simulink model "Drone_Simulation"  (R2020a)
settings: Solver=ode1  StartTime=0.0  StopTime=50  FixedStep=1e-3
values from neighbouring files (symbols this model uses):
  AeEMSC = 1    [Qball_X8_Model.m]
  alpha1TDDBSC = 1    [Qball_X8_Model.m]    (also in ReliabilityModel_Script.m = 0.7)
  bBNG = 1.2    [ReliabilityModel_Script.m]
  bEMSC = 1    [Qball_X8_Model.m]
  bEVCAP = 1    [Qball_X8_Model.m]    (also in ReliabilityModel_Script.m = 1.1)
  BNG_Motor1 = 0.8    [ReliabilityModel_Script.m]
  BNG_Motor2 = 1    [ReliabilityModel_Script.m]
  BNG_Motor3 = 1    [ReliabilityModel_Script.m]
  BNG_Motor4 = 1    [ReliabilityModel_Script.m]
  BNG_Motor5 = 1    [ReliabilityModel_Script.m]
  BNG_Motor6 = 1    [ReliabilityModel_Script.m]
  bp = 0.001    [ControlLawsScript.m]    (also in ControlLaws_Script.m)
  bq = 0.001    [ControlLawsScript.m]    (also in ControlLaws_Script.m)
  br = 0.001    [ControlLawsScript.m]    (also in ControlLaws_Script.m)
  bTDDBSC = 1    [Qball_X8_Model.m]    (also in ReliabilityModel_Script.m = 1.1)
  bWDG = 1    [Qball_X8_Model.m]    (also in ReliabilityModel_Script.m = 1.1)
  C_A = [     k_T           k_T          k_T                k_T          k_T         k_T ... (first row only)    [ControlLawsScript.m]    (also in ControlLaws_Script.m)
  C_mot = 1    [Qball_X8_Model.m]    (also in ReliabilityModel_Script.m = 17.46)
  C_th_esc = 1    [Qball_X8_Model.m]    (also in ReliabilityModel_Script.m = 1.67)
  CAPEV_Motor1 = 0.8    [ReliabilityModel_Script.m]
  CAPEV_Motor2 = 1    [ReliabilityModel_Script.m]
  CAPEV_Motor3 = 1    [ReliabilityModel_Script.m]
  CAPEV_Motor4 = 1    [ReliabilityModel_Script.m]
  CAPEV_Motor5 = 1    [ReliabilityModel_Script.m]
  CAPEV_Motor6 = 1    [ReliabilityModel_Script.m]
  cdx = cx*m    (= 17.4057414746)    [ControlLawsScript.m]    (also in ControlLaws_Script.m)
  cdy = cy*m    (= 17.4057414746)    [ControlLawsScript.m]    (also in ControlLaws_Script.m)
  cdz = cz*m    (= 17.4057414746)    [ControlLawsScript.m]    (also in ControlLaws_Script.m)
  EaEMSC = 1    [Qball_X8_Model.m]
  EaEVCAP = 1    [Qball_X8_Model.m]    (also in ReliabilityModel_Script.m = 0.94)
  EalphaTDDBSC = 1    [Qball_X8_Model.m]    (also in ReliabilityModel_Script.m = 0.7)
  EaTDDBSC = 1    [Qball_X8_Model.m]    (also in ReliabilityModel_Script.m = 0.7)
  EaWDG = 1    [Qball_X8_Model.m]    (also in ReliabilityModel_Script.m = 0.5)
  g = 9.80665    [ControlLawsScript.m]    (also in ControlLaws_Script.m; Qball_X8_Model.m = 9.87)
  JrefEMSC = 1    [Qball_X8_Model.m]
  Jz = 0.15887270137511    (= 0.158872701375)    [ControlLawsScript.m]    (also in ControlLaws_Script.m)
  k_b = 1    [Qball_X8_Model.m]    (also in ReliabilityModel_Script.m = -21.8546)
  Kp = (Jx/Tc)-bp    (= 4.11390529802)    [ControlLawsScript.m]    (also in ControlLaws_Script.m)
  Kp2 = Jx*((4/ts))*((-4/ts)+((bp+Kp)/Jx))/Kp    (= 6.72163348437)    [ControlLawsScript.m]    (also in ControlLaws_Script.m)
  Kq = (Jy/Tc)-bq    (= 4.12186008142)    [ControlLawsScript.m]    (also in ControlLaws_Script.m)
  Kq2 = Jy*((4/ts))*((-4/ts)+((bq+Kq)/Jy))/Kq    (= 6.72163033191)    [ControlLawsScript.m]    (also in ControlLaws_Script.m)
  Kr = (Jz/(tsy/25))-br    (= 7.94263506876)    [ControlLawsScript.m]    (also in ControlLaws_Script.m)
  Kr2 = Jz*((4/tsy))*((-4/tsy)+((br+Kr)/Jz))/Kr    (= 6.72084606682)    [ControlLawsScript.m]    (also in ControlLaws_Script.m)
  kv = 1/930    (= 0.0010752688172)    [StingerScript.m]
  Kx = abs(Kx)    [ControlLawsScript.m]    (also in ControlLaws_Script.m)
  Ky = abs(Ky)    [ControlLawsScript.m]    (also in ControlLaws_Script.m)
  Kz = (m/Tcz)-cz    (= 38.5143536865)    [ControlLawsScript.m]    (also in ControlLaws_Script.m)
  Kz2 = m*((4/tsz))*((-4/tsz)+((cz+Kz)/m))/Kz    (= 1.89810050529)    [ControlLawsScript.m]    (also in ControlLaws_Script.m)
  LnomEMSC = 1    [Qball_X8_Model.m]
  LnomEVCAP = 1    [Qball_X8_Model.m]    (also in ReliabilityModel_Script.m = 10800000)
  LnomTDDBSC = 1    [Qball_X8_Model.m]    (also in ReliabilityModel_Script.m = 9997200)
  LnomWDG = 1    [Qball_X8_Model.m]    (also in ReliabilityModel_Script.m = 72000000)
  m = 3.4811482949175    (= 3.48114829492)    [ControlLawsScript.m]    (also in ControlLaws_Script.m; Qball_X8_Model.m = 1.45)
  max_yaw_moment = k_y*hov_thrust/k_T    (= 0.323744079512)    [ControlLawsScript.m]    (also in ControlLaws_Script.m = 0.57666914163)
  NEMSC = 1    [Qball_X8_Model.m]
  nEVCAP = 1    [Qball_X8_Model.m]    (also in ReliabilityModel_Script.m)
  pconst = 2    [Qball_X8_Model.m]    (also in ReliabilityModel_Script.m)
  pitch_angle_limit = 32/R2D    (= 0.558505360638)    [ControlLawsScript.m]    (also in ControlLaws_Script.m)
  R2D = 180/pi    (= 57.2957795131)    [ControlLawsScript.m]    (also in ControlLaws_Script.m)
  R_th_esc = 1    [Qball_X8_Model.m]    (also in ReliabilityModel_Script.m = 5.14)
  R_th_mot = 1    [Qball_X8_Model.m]    (also in ReliabilityModel_Script.m = 8.59)
  Re = 0.008    [Qball_X8_Model.m]    (also in ReliabilityModel_Script.m)
  roll_angle_limit = 32/R2D    (= 0.558505360638)    [ControlLawsScript.m]    (also in ControlLaws_Script.m)
  RrefBNG = 0.9    [ReliabilityModel_Script.m]
  RrefEMSC = 1    [Qball_X8_Model.m]
  RrefEVCAP = 1    [Qball_X8_Model.m]    (also in ReliabilityModel_Script.m = 0.9)
  RrefTDDBSC = 1    [Qball_X8_Model.m]    (also in ReliabilityModel_Script.m = 0.37)
  RrefWDG = 1    [Qball_X8_Model.m]    (also in ReliabilityModel_Script.m = 0.98)
  SCTDDB_Motor1 = 0.8    [ReliabilityModel_Script.m]
  SCTDDB_Motor2 = 1    [ReliabilityModel_Script.m]
  SCTDDB_Motor3 = 1    [ReliabilityModel_Script.m]
  SCTDDB_Motor4 = 1    [ReliabilityModel_Script.m]
  SCTDDB_Motor5 = 1    [ReliabilityModel_Script.m]
  SCTDDB_Motor6 = 1    [ReliabilityModel_Script.m]
  T_amb = 1    [Qball_X8_Model.m]    (also in ReliabilityModel_Script.m = 20)
  T_amb_mot = 1    [Qball_X8_Model.m]    (also in ReliabilityModel_Script.m = 20)
  t_D_SCTDDB = 30    [ReliabilityModel_Script.m]
  TrefEMSC = 1    [Qball_X8_Model.m]
  TrefEVCAP = 1    [Qball_X8_Model.m]    (also in ReliabilityModel_Script.m = 105)
  TrefTDDBSC = 1    [Qball_X8_Model.m]    (also in ReliabilityModel_Script.m = 150)
  TrefWDG = 1    [Qball_X8_Model.m]    (also in ReliabilityModel_Script.m = 40)
  Ub = 12    [Qball_X8_Model.m]    (also in ReliabilityModel_Script.m)
  VmaxEVCAP = 1    [Qball_X8_Model.m]    (also in ReliabilityModel_Script.m = 35)
  VnomEVCAP = 1    [Qball_X8_Model.m]    (also in ReliabilityModel_Script.m = 35)
  WDG_Motor1 = 0.8    [ReliabilityModel_Script.m]
  WDG_Motor2 = 1    [ReliabilityModel_Script.m]
  WDG_Motor3 = 1    [ReliabilityModel_Script.m]
  WDG_Motor4 = 1    [ReliabilityModel_Script.m]
  WDG_Motor5 = 1    [ReliabilityModel_Script.m]
  WDG_Motor6 = 1    [ReliabilityModel_Script.m]
  z_x = cx    (= 5)    [ControlLawsScript.m]    (also in ControlLaws_Script.m)
  z_y = cy    (= 5)    [ControlLawsScript.m]    (also in ControlLaws_Script.m)
undefined symbols (not defined in the file or in its folder): FuselageContactForces, LeftAftArm, LeftAftSkid, LeftArm, LeftFrontArm, LeftFrontSkid, LeftSideContactForces, Lower, missionPlanX, missionPlanY, missionPlanYaw, missionPlanZ, Newton, Raphson, RightAftArm, RightAftSkid, RightArm, RightFrontArm, RightFrontSkid, RightSideContactForces, SkidsContactForces, timeConstant, Upper, X, Y, Z
libraries: sm_lib x90, nesl_utility x78, fl_lib x61, ee_lib x19, dspinverses x1, dspmtrx3 x1
(part 2 of 5)

== system Drone_Simulation/CONTROL ALLOCATION/Reliability Observer (SCTDDB)1 ==
  T_IN : Inport
  V_ESC_OUT : Inport  Port=2
  Cumulative Aging VTDDB : Subsystem
  LambdaTDDB : Subsystem
  ReliabilityTDDB : Subsystem
  VrefTDDB : Subsystem
  R_RT_SCTDDB : Outport
  LambdaSCTDDB : Outport  Port=2
  wires:
  V_ESC_OUT/1 -> Cumulative Aging VTDDB/2(V_ESC_OUT)
  LambdaTDDB/1(Out1) -> LambdaSCTDDB/1
  ReliabilityTDDB/1(Out1) -> R_RT_SCTDDB/1
  Cumulative Aging VTDDB/1(Out1) -> LambdaTDDB/1(In1), ReliabilityTDDB/1(In1)
  VrefTDDB/1(Out1) -> LambdaTDDB/2(In2), ReliabilityTDDB/2(In2)
  T_IN/1 -> Cumulative Aging VTDDB/1(T_IN)

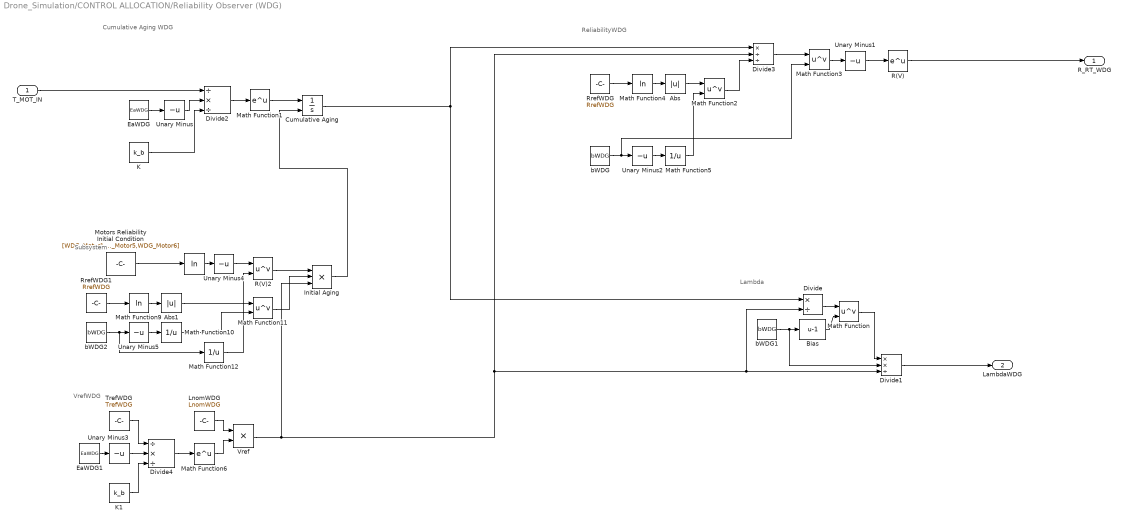
== system Drone_Simulation/CONTROL ALLOCATION/Reliability Observer (WDG) ==
  note: Lambda
  note: ReliabilityWDG
  note: VrefWDG
  note: Cumulative Aging WDG
  note: Subsystem
  T_MOT_IN : Inport
  " " : Math  Operator=log  SaturateOnIntegerOverflow=on
  Abs : Abs
  Abs1 : Abs
  Bias : Bias  Bias=-1
  Cumulative Aging : Integrator  InitialConditionSource=external
  Divide : Product  Inputs=*/
  Divide1 : Product  Inputs=**/
  Divide2 : Product  Inputs=/*/
  Divide3 : Product  Inputs=*//
  Divide4 : Product  Inputs=/*/
  EaWDG : Constant  Value=EaWDG
  EaWDG1 : Constant  Value=EaWDG
  Initial Aging : Product  Inputs=3
  K : Constant  Value=k_b
  K1 : Constant  Value=k_b
  LnomWDG : Constant  Value=LnomWDG
  Math Function{,2..3,11} (4 alike) : Math  Operator=pow  SaturateOnIntegerOverflow=on
  Math Function1 : Math  SaturateOnIntegerOverflow=on
  Math Function10 : Math  Operator=reciprocal  SaturateOnIntegerOverflow=on
  Math Function12 : Math  Operator=reciprocal  SaturateOnIntegerOverflow=on
  Math Function4 : Math  Operator=log  SaturateOnIntegerOverflow=on
  Math Function5 : Math  Operator=reciprocal  SaturateOnIntegerOverflow=on
  Math Function6 : Math  SaturateOnIntegerOverflow=on
  Math Function9 : Math  Operator=log  SaturateOnIntegerOverflow=on
  Motors Reliability Initial Condition : Constant  Value=[WDG_Motor1,WDG_Motor2,WDG_Motor3,WDG_Motor4,WDG_Motor5,WDG_Motor6]
  R(V) : Math  SaturateOnIntegerOverflow=on
  R(V)2 : Math  Operator=pow  SaturateOnIntegerOverflow=on
  RrefWDG : Constant  Value=RrefWDG
  RrefWDG1 : Constant  Value=RrefWDG
  TrefWDG : Constant  Value=TrefWDG
  Unary Minus{,1..5} (6 alike) : UnaryMinus
  Vref : Product
  bWDG : Constant  Value=bWDG
  bWDG1 : Constant  Value=bWDG
  bWDG2 : Constant  Value=bWDG
  R_RT_WDG : Outport
  LambdaWDG : Outport  Port=2
  wires:
  Divide1/1 -> LambdaWDG/1
  R(V)/1 -> R_RT_WDG/1
  T_MOT_IN/1 -> Divide2/1
  Unary Minus/1 -> Divide2/2
  Divide2/1 -> Math Function1/1
  K/1 -> Divide2/3
  EaWDG/1 -> Unary Minus/1
  Math Function1/1 -> Cumulative Aging/1
  TrefWDG/1 -> Divide4/1
  Divide4/1 -> Math Function6/1
  Math Function6/1 -> Vref/2
  LnomWDG/1 -> Vref/1
  K1/1 -> Divide4/3
  Unary Minus3/1 -> Divide4/2
  EaWDG1/1 -> Unary Minus3/1
  Unary Minus2/1 -> Math Function5/1
  Math Function2/1 -> Divide3/3
  RrefWDG/1 -> Math Function4/1
  Math Function5/1 -> Math Function2/2
  Math Function3/1 -> Unary Minus1/1
  bWDG/1 -> Math Function3/2, Unary Minus2/1
  Unary Minus1/1 -> R(V)/1
  Math Function4/1 -> Abs/1
  Abs/1 -> Math Function2/1
  Divide3/1 -> Math Function3/1
  Cumulative Aging/1 -> Divide3/1, Divide/1
  Divide/1 -> Math Function/1
  bWDG1/1 -> Divide1/2, Bias/1
  Math Function/1 -> Divide1/1
  Bias/1 -> Math Function/2
  Vref/1 -> Divide3/2, Divide/2, Divide1/3, Initial Aging/3
  Initial Aging/1 -> Cumulative Aging/2
  Math Function12/1 -> R(V)2/2
  Math Function10/1 -> Math Function11/2
  R(V)2/1 -> Initial Aging/1
  Math Function9/1 -> Abs1/1
  Abs1/1 -> Math Function11/1
  RrefWDG1/1 -> Math Function9/1
  bWDG2/1 -> Math Function12/1, Unary Minus5/1
  " "/1 -> Unary Minus4/1
  Unary Minus4/1 -> R(V)2/1
  Motors Reliability Initial Condition/1 -> " "/1
  Math Function11/1 -> Initial Aging/2
  Unary Minus5/1 -> Math Function10/1

== system Drone_Simulation/CONTROL ALLOCATION/Reliability Observer (WDG)1 ==
  T_MOT_IN : Inport
  Cumulative Aging WDG : Subsystem
  Display : Display
  Lambda : Subsystem
  ReliabilityWDG : Subsystem
  VrefWDG : Subsystem
  R_RT_WDG : Outport
  LambdaWDG : Outport  Port=2
  wires:
  ReliabilityWDG/1(Out1) -> R_RT_WDG/1
  T_MOT_IN/1 -> Cumulative Aging WDG/1(In1)
  Cumulative Aging WDG/1(Out1) -> ReliabilityWDG/1(In1), Lambda/1(In1), Display/1
  VrefWDG/1(Out1) -> ReliabilityWDG/2(In2), Lambda/2(In2)
  Lambda/1(Out1) -> LambdaWDG/1

== system Drone_Simulation/CONTROL ALLOCATION/Thermal Model (ESC)2 ==
  note: Will update, temporary values ->
  V_ESC_in (V) : Inport  PortDimensions=6
  I_ESC_in (A) : Inport  Port=2  PortDimensions=6
  V_ESC_OUT : Inport  Port=3
  I_ESC_OUT : Inport  Port=4
  Demux : Demux  Outputs=6
  Display : Display
  Mux : Mux  Inputs=6
      settings: DisplayOption=signals
  Product : Product
  Product1 : Product
  Product2 : Product
  R_th_esc : Constant  Value=[R_th_esc;R_th_esc;R_th_esc;R_th_esc;R_th_esc;R_th_esc]
  Saturation : Saturate  UpperLimit=400  LowerLimit=T_amb
  Subtract : Sum  Inputs=+-
  Subtract1 : Sum
  T_amb : Constant  Value=[T_amb;T_amb;T_amb;T_amb;T_amb;T_amb]
  Transfer Fcn{,1..5} (6 alike) : TransferFcn  Denominator=[R_th_esc*C_th_esc 1]
  T_ESC_IN : Outport
  wires:
  V_ESC_in (V)/1 -> Product/1
  I_ESC_in (A)/1 -> Product/2
  Product/1 -> Subtract/1
  Product2/1 -> Subtract/2
  Subtract/1 -> Product1/1
  R_th_esc/1 -> Product1/2
  Product1/1 -> Subtract1/1
  V_ESC_OUT/1 -> Product2/1
  I_ESC_OUT/1 -> Product2/2
  Subtract1/1 -> Demux/1
  Transfer Fcn5/1 -> Mux/6
  Transfer Fcn1/1 -> Mux/2
  Transfer Fcn4/1 -> Mux/5
  Transfer Fcn/1 -> Mux/1
  Transfer Fcn3/1 -> Mux/4
  Demux/1 -> Transfer Fcn/1
  Transfer Fcn2/1 -> Mux/3
  Demux/3 -> Transfer Fcn2/1
  Demux/6 -> Transfer Fcn5/1
  Demux/5 -> Transfer Fcn4/1
  Demux/4 -> Transfer Fcn3/1
  Demux/2 -> Transfer Fcn1/1
  T_amb/1 -> Subtract1/2
  Saturation/1 -> Display/1, T_ESC_IN/1
  Mux/1 -> Saturation/1

== system Drone_Simulation/CONTROL ALLOCATION/Thermal Model (Motor)2 ==
  Torque : Inport  PortDimensions=6
  RPM : Inport  Port=2  PortDimensions=6
  V_ESC_OUT : Inport  Port=3  PortDimensions=6
  I_ESC_OUT : Inport  Port=4  PortDimensions=6
  Delay : Delay
  Demux : Demux  Outputs=6
  Display : Display
  Display1 : Display
  Display2 : Display
  Gain : Gain  Gain=pi/180
  Mux : Mux  Inputs=6
  Product : Product
  Product1 : Product
  Product2 : Product
  R_th_mot : Constant  Value=[R_th_mot;R_th_mot;R_th_mot;R_th_mot;R_th_mot;R_th_mot]
  Saturation : Saturate  UpperLimit=400  LowerLimit=T_amb_mot
  Subtract : Sum  Inputs=+-
  Subtract1 : Sum
  T_amb_mot : Constant  Value=[T_amb_mot;T_amb_mot;T_amb_mot;T_amb_mot;T_amb_mot;T_amb_mot]
  Transfer Fcn{,1..5} (6 alike) : TransferFcn  Denominator=[R_th_mot*C_mot 1]
  T_MOT_IN : Outport  PortDimensions=6
  wires:
  Subtract/1 -> Product1/1
  R_th_mot/1 -> Product1/2
  Product1/1 -> Subtract1/1, Display/1
  T_amb_mot/1 -> Display1/1, Subtract1/2
  Product2/1 -> Subtract/1
  Product/1 -> Subtract/2
  Torque/1 -> Product/1
  I_ESC_OUT/1 -> Product2/2
  V_ESC_OUT/1 -> Delay/1
  Subtract1/1 -> Demux/1
  Demux/1 -> Transfer Fcn/1
  Demux/2 -> Transfer Fcn1/1
  Demux/4 -> Transfer Fcn3/1
  Demux/3 -> Transfer Fcn2/1
  Demux/5 -> Transfer Fcn4/1
  Demux/6 -> Transfer Fcn5/1
  Transfer Fcn/1 -> Mux/1
  Transfer Fcn1/1 -> Mux/2
  Transfer Fcn3/1 -> Mux/4
  Transfer Fcn4/1 -> Mux/5
  Mux/1 -> Saturation/1, Display2/1
  Gain/1 -> Product/2
  RPM/1 -> Gain/1
  Transfer Fcn2/1 -> Mux/3
  Transfer Fcn5/1 -> Mux/6
  Delay/1 -> Product2/1
  Saturation/1 -> T_MOT_IN/1

== system Drone_Simulation/PLANT MODEL/BODY ==
  Lower Body : sm_lib/Body Elements/File Solid  ExtGeomFileName=STL files\LowerBody.stl  UnitType=Custom  ExtGeomFileUnits=mm  StepReaderType=HEX  ExportConvexHullGeometry=on  InertiaType=CalculateFromGeometry  Mass=1.038628  MassUnits=kg  CenterOfMass=[0, 0, -1.64462e-2]  CenterOfMassUnits=m  MomentsOfInertia=[5.66226e-3 5.662277e-3 1.11925e-2]  MomentsOfInertiaUnits=kg*m^2  ProductsOfInertia=[0 0 6.64514e-10]  ProductsOfInertiaUnits=kg*m^2  BasedOnType=Density  Density=rho  DensityUnits=kg/m^3  DoExposeReferenceFrame=on  SerializedFrames=<Frames/>  GraphicType=FromGeometry  MarkerShape=Sphere  MarkerSize=10  GraphicVisPropType=SimpleVisualProperties  GraphicDiffuseColor=rgb  GraphicSpecularColor=[0.5 0.5 0.5 1.0]  GraphicAmbientColor=[0.15 0.15 0.15 1.0]  GraphicEmissiveColor=[0.0 0.0 0.0 1.0]  GraphicShininess=75  GraphicOpacity=op
  SKIDS : Subsystem  mask{rho2=788, rgb2=[1 1 1], op2=1}
      mask prompts: rho2 "Density of Skid (kg/m^3)"; rgb2 "Color of Skid [R G B]"; op2 "Opacity of Skid (0-1)"
      mask Display: image('$imagefile'); % Use "Edit Image" on toolstrip to change.
  Simscape Bus : SimscapeBus  HierarchyStrings=Upper;Lower
  Upper Body : sm_lib/Body Elements/File Solid  ExtGeomFileName=STL files\UpperBody.stl  UnitType=Custom  ExtGeomFileUnits=mm  StepReaderType=HEX  ExportConvexHullGeometry=on  InertiaType=CalculateFromGeometry  Mass=1.05986327  MassUnits=kg  CenterOfMass=[0 0 1.6454e-2]  CenterOfMassUnits=m  MomentsOfInertia=[5.7148e-3 5.6834e-3 1.12655e-2]  MomentsOfInertiaUnits=kg*m^2  ProductsOfInertia=[0 0 6.7805e-10]  ProductsOfInertiaUnits=kg*m^2  BasedOnType=Density  Density=rho  DensityUnits=kg/m^3  DoExposeReferenceFrame=on  SerializedFrames=<Frames/>  GraphicType=FromGeometry  MarkerShape=Sphere  MarkerSize=10  GraphicVisPropType=SimpleVisualProperties  GraphicDiffuseColor=rgb  GraphicSpecularColor=[0.5 0.5 0.5 1.0]  GraphicAmbientColor=[0.15 0.15 0.15 1.0]  GraphicEmissiveColor=[0.0 0.0 0.0 1.0]  GraphicShininess=75  GraphicOpacity=op
  Contact : PMIOPort  Side=Left
  Plant : PMIOPort  Port=2  Side=Right
  Contact1 : PMIOPort  Port=3  Side=Left
  connections:
  Upper Body/LConn1 -- Simscape Bus/LConn1
  Upper Body/RConn1 -- Lower Body/RConn1 -- Plant/RConn1 -- SKIDS/LConn2
  Contact/RConn1 -- Simscape Bus/RConn1
  Simscape Bus/LConn2 -- Lower Body/LConn1
  Contact1/RConn1 -- SKIDS/LConn1

== system Drone_Simulation/PLANT MODEL/CONTACT FORCES ==
  Left Contact Arms : SimscapeBus  HierarchyStrings=LeftFrontArm;LeftArm;LeftAftArm
  Right Contact Arms : SimscapeBus  HierarchyStrings=RightFrontArm;RightArm;RightAftArm
  Right Contact Skids : SimscapeBus  HierarchyStrings=LeftAftSkid;LeftFrontSkid;RightFrontSkid;RightAftSkid
  Simscape Bus : SimscapeBus  HierarchyStrings=FuselageContactForces;LeftSideContactForces;RightSideContactForces;SkidsContactForces
  Simscape Bus1 : SimscapeBus  HierarchyStrings=Upper;Lower
  Spatial Contact Force{,1..11} (12 alike) : sm_lib/Forces and Torques/Spatial Contact Force  CoefficientOfDynamicFriction=mud  CoefficientOfStaticFriction=mus  NormalDamping=b  NormalDampingUnits=N/(m/s)  NormalStiffness=st  NormalStiffnessUnits=N/m  FrictionalCriticalVelocity=vcr  FrictionalCriticalVelocityUnits=m/s  ZeroCrossDetectContactStartAndEnd=off  SenseFrictionalForceMagnitude=off  SenseNormalForceMagnitude=off  SenseSeparationDistance=off  NormalTransitionRegionWidth=trans  NormalTransitionRegionWidthUnits=m  FrictionType=SmoothStickSlip
  GC : PMIOPort  Side=Right
  Contact Forces : PMIOPort  Port=2  Side=Right
  connections:
  Spatial Contact Force/RConn1 -- Spatial Contact Force9/RConn1 -- GC/RConn1 -- Spatial Contact Force1/RConn1 -- Spatial Contact Force2/RConn1 -- Spatial Contact Force3/RConn1 -- Spatial Contact Force4/RConn1 -- Spatial Contact Force5/RConn1 -- Spatial Contact Force6/RConn1 -- Spatial Contact Force11/RConn1 -- Spatial Contact Force10/RConn1 -- Spatial Contact Force8/RConn1 -- Spatial Contact Force7/RConn1
  Right Contact Arms/LConn3 -- Spatial Contact Force6/LConn1
  Right Contact Arms/LConn2 -- Spatial Contact Force5/LConn1
  Right Contact Arms/LConn1 -- Spatial Contact Force4/LConn1
  Left Contact Arms/LConn2 -- Spatial Contact Force2/LConn1
  Spatial Contact Force1/LConn1 -- Left Contact Arms/LConn1
  Left Contact Arms/LConn3 -- Spatial Contact Force3/LConn1
  Right Contact Skids/LConn1 -- Spatial Contact Force11/LConn1
  Right Contact Skids/LConn2 -- Spatial Contact Force10/LConn1
  Spatial Contact Force8/LConn1 -- Right Contact Skids/LConn3
  Right Contact Skids/LConn4 -- Spatial Contact Force7/LConn1
  Simscape Bus/LConn2 -- Left Contact Arms/RConn1
  Simscape Bus/LConn3 -- Right Contact Arms/RConn1
  Simscape Bus/LConn4 -- Right Contact Skids/RConn1
  Contact Forces/RConn1 -- Simscape Bus/RConn1
  Simscape Bus1/RConn1 -- Simscape Bus/LConn1
  Spatial Contact Force/LConn1 -- Simscape Bus1/LConn2
  Spatial Contact Force9/LConn1 -- Simscape Bus1/LConn1

== system Drone_Simulation/PLANT MODEL/DRAG FORCES ==
  note: Drag Constants
  External Force and Torque : sm_lib/Forces and Torques/External Force and Torque  ForceResolutionFrame=AttachedFrame  EnableForceX=on  EnableForceY=on  EnableForceZ=on  EnableForce=off  TorqueResolutionFrame=AttachedFrame  EnableTorqueX=on  EnableTorqueY=on  EnableTorqueZ=on  EnableTorque=off
  Gain15 : Gain  Gain=-cdx
  Gain16 : Gain  Gain=-cdy
  Gain17 : Gain  Gain=-cdz
  Gain18 : Gain  Gain=-bq
  Gain19 : Gain  Gain=0
  Gain20 : Gain  Gain=bp
  Simulink-PS Converter{,1..5} (6 alike) : nesl_utility/Simulink-PS Converter  PhysicalDomain=network_engine_domain  SubClassName=ps_input  LeftPortType=input  RightPortType=output  PseudoPeriodic=off  Frequencies=[]  NoiseDistribution=none  NoiseParameters=[]  Unit=1  AffineConversion=off  FilteringAndDerivatives=provide  SimscapeFilterOrder=1  InputFilterTimeConstant=0.001  UdotUserProvided=0
  Model : PMIOPort  Side=Right
  wires:
  Gain20/1 -> Simulink-PS Converter/1  "tx"
  Gain17/1 -> Simulink-PS Converter3/1  "fz"
  Gain15/1 -> Simulink-PS Converter5/1  "fx"
  Gain16/1 -> Simulink-PS Converter4/1  "fy"
  Gain18/1 -> Simulink-PS Converter1/1  "ty"
  Gain19/1 -> Simulink-PS Converter2/1  "tz"
  [DZ] -> Gain17/1
  [DY] -> Gain16/1
  [DX] -> Gain15/1
  [rollAngleSpeed] -> Gain20/1
  [pitchAngleSpeed] -> Gain18/1
  [yawAngleSpeed] -> Gain19/1
  connections:
  Simulink-PS Converter4/RConn1 -- External Force and Torque/LConn2
  Simulink-PS Converter5/RConn1 -- External Force and Torque/LConn1
  Simulink-PS Converter2/RConn1 -- External Force and Torque/LConn6
  Simulink-PS Converter/RConn1 -- External Force and Torque/LConn4
  Simulink-PS Converter1/RConn1 -- External Force and Torque/LConn5
  Simulink-PS Converter3/RConn1 -- External Force and Torque/LConn3
  Model/RConn1 -- External Force and Torque/RConn1

== system Drone_Simulation/PLANT MODEL/ELECTRIC SYSTEM ==
  Battery 1 (Table-Based)1 : ee_lib/Sources/Battery (Table-Based)  Commented=on  SOC_vec=[0,0.05,0.1,0.15,0.2,0.25,0.3,0.35,0.4,0.45,0.5,0.55,0.6,0.65,0.7,0.75,0.8,0.85,0.9,0.95,1]  T_dependence=ee.enum.temperature_dependence.no  T_vec=[273.15, 298.15, 323.15] K  V0_mat=[3.2, 3.1, 3.14; 3.25, 3.27, 3.3; 3.28, 3.31, 3.34; 3.33, 3.5, 3.59] V  V0_vec=[0,12,13,13.4,13.62,13.75,13.85,13.91,13.95,14,14,14,14,14,14,14,14,14,14,14.6,16.8] V  R0_mat=[.03, .015, .002; .04, .017, .008; .039, .012, .006; .027, .013, .021] Ohm  R0_vec=[0.014,0.014,0.014,0.014,0.014,0.014,0.014,0.014,0.014,0.014,0.014,0.014,0.014,0.014,0.014,0.014,0.014,0.014,0.014,0.014,0.014] Ohm  AH_vec=[2.9, 4.1, 4.2] hr*A  AH=5.2 hr*A  prm_leak=ee.enum.battery.prm_leak.disabled  Rleak_vec=[8000, 7000, 6000] Ohm  Rleak=7e3 Ohm  extrapolation_option=ee.enum.extrapolation.nearest  prm_dyn=ee.enum.battery.prm_dyn.off  R1_mat=[.089, .076, .01; .042, .022, .099; .019, .007, .002; .051, .043, .029] Ohm  R1_vec=[.076, .022, .007, .043] Ohm  tau1_mat=[44, 148, 235; 93, 110, 1000; 19, 27, 133; .5, 22, 3] s  tau1_vec=[148, 110, 27, 22] s  R2_mat=[.014, .382, .407; .028, .006, .007; .014, .007, .006; .333, .956, .912] Ohm  R2_vec=[.382, .006, .007, .956] Ohm  tau2_mat=[1, 44, 5644; 11, 24, 506; 2, 14, 330; 3310, 13419, 30216] s  tau2_vec=[44, 24, 14, 13419] s  R3_mat=[.014, .382, .407; .028, .006, .007; .014, .007, .006; .333, .956, .912] Ohm  R3_vec=[.382, .006, .007, .956] Ohm  tau3_mat=[1, 44, 5644; 11, 24, 506; 2, 14, 330; 3310, 13419, 30216] s  tau3_vec=[44, 24, 14, 13419] s  R4_mat=[.014, .382, .407; .028, .006, .007; .014, .007, .006; .333, .956, .912] Ohm  R4_vec=[.382, .006, .007, .956] Ohm  tau4_mat=[1, 44, 5644; 11, 24, 506; 2, 14, 330; 3310, 13419, 30216] s  tau4_vec=[44, 24, 14, 13419] s  R5_mat=[.014, .382, .407; .028, .006, .007; .014, .007, .006; .333, .956, .912] Ohm  R5_vec=[.382, .006, .007, .956] Ohm  tau5_mat=[1, 44, 5644; 11, 24, 506; 2, 14, 330; 3310, 13419, 30216] s  tau5_vec=[44, 24, 14, 13419] s  prm_fade=ee.enum.battery.prm_fade.equations  N0=100  dV0=0  dR0=0  dAH=0  dRleak=0  dR1=0  dR2=0  dR3=0  dR4=0  dR5=0  N0vec=[100, 200, 300]  Tfadevec=[298.15, 323.15] K  dV0vec=[0, 0, 0]  dR0vec=[0, 0, 0]  dAHvec=[0, 0, 0]  dRleakvec=[0, 0, 0]  dR1vec=[0, 0, 0]  dR2vec=[0, 0, 0]  dR3vec=[0, 0, 0]  dR4vec=[0, 0, 0]  dR5vec=[0, 0, 0]  dV0mat=[0, 0; 0, 0; 0, 0]  dR0mat=[0, 0; 0, 0; 0, 0]  dAHmat=[0, 0; 0, 0; 0, 0]  dRleakmat=[0, 0; 0, 0; 0, 0]  dR1mat=[0, 0; 0, 0; 0, 0]  dR2mat=[0, 0; 0, 0; 0, 0]  dR3mat=[0, 0; 0, 0; 0, 0]  dR4mat=[0, 0; 0, 0; 0, 0]  dR5mat=[0, 0; 0, 0; 0, 0]  temperature=298.15 K  i_specify=off  i_priority=None  i=0 A  i_nominal_specify=off  i_nominal_unit=A  i_nominal_value=1  v_specify=off  v_priority=None  v=0 V  v_nominal_specify=off  v_nominal_unit=V  v_nominal_value=1  stateOfCharge_specify=on  stateOfCharge_priority=High  stateOfCharge=In_SOC_Bat1  stateOfCharge_nominal_specify=off  stateOfCharge_nominal_unit=1  stateOfCharge_nominal_value=1  num_cycles_specify=off  num_cycles_priority=High  num_cycles=0  num_cycles_nominal_specify=off  num_cycles_nominal_unit=1  num_cycles_nominal_value=1  thermal_mass=30000 J/K  temperature_specify=off  temperature_priority=High  temperature_nominal_specify=off  temperature_nominal_unit=K  temperature_nominal_value=1
      settings: SourceProductBaseCode=PS  InternalSimscapePortConfiguration="{\"Bottom\":[],\"Left\":[{\"id\":\"p\",\"label\":\"+\",\"type\":\"foundation.electrical.electrical\"}],\"Right\":[{\"id\":\"n\",\"label\":\"-\",\"type\":\"foundation.electrical.electrical\"}],\"Top\":[]}"
  Battery 1 (Model based) : fl_lib/Electrical/Electrical Sources/Controlled Voltage Source
  Battery 2 (Model based) : fl_lib/Electrical/Electrical Sources/Controlled Voltage Source
  Current Sensor 1 : fl_lib/Electrical/Electrical Sensors/Current Sensor
  Current Sensor 2 : fl_lib/Electrical/Electrical Sensors/Current Sensor
  Display : Display
  Ground : fl_lib/Electrical/Electrical Elements/Electrical Reference
  Motor 1 : Subsystem
      settings: PortSchema="{\"entries\":[{\"content\":{\"sides\":[{\"content\":{},\"type\":\"ConnectorPlacement.EquallySpacedRectSide\",\"uuid\":\"08d870a7-e796-404b-a5f6-b37f0e33392d\"},{\"content\":{\"side\":\"RIGHT\"},\"type\":\"ConnectorPlacement.EquallySpacedRectSide\",\"uuid\":\"df51a617-9ca1-4f8a-b830-66ef9da37eb2\"},{\"content\":{\"connectorIds\":[\"LConn1\"],\"side\":\"TOP\"},\"type\":\"ConnectorPlacement.EquallySpacedRectSide\",\"uuid\":\"0bf9cc2e-db18-4280-a0b6-874c36a8e80d\"},{\"content\":{\"connectorIds\":[\"RConn1\"],\"side\":\"BOTTOM\"},\"type\":\"ConnectorPlacement.EquallySpacedRectSide\",\"uuid\":\"837a9097-ff08-480d-b5bf-68b48d68c34c\"}]},\"type\":\"ConnectorPlacement.EquallySpacedConnector\",\"uuid\":\"55e23bf7-a9a7-40c2-835c-208173f510f1\"}],\"packageUris\":[\"http://schema.mathworks.com/mf0/Connector/R2020b\"],\"version\":\"1.0\"}"
      mask Display: image('$imagefile'); % Use "Edit Image" on toolstrip to change.
  Motor 2 : Subsystem
      settings: PortSchema="{\"entries\":[{\"content\":{\"sides\":[{\"content\":{},\"type\":\"ConnectorPlacement.EquallySpacedRectSide\",\"uuid\":\"be0e671a-e613-444c-b8e2-6f7a2adfd701\"},{\"content\":{\"side\":\"RIGHT\"},\"type\":\"ConnectorPlacement.EquallySpacedRectSide\",\"uuid\":\"98a92d25-e065-434b-83fd-1db07c9786c9\"},{\"content\":{\"connectorIds\":[\"LConn1\",\"LConn2\"],\"side\":\"TOP\"},\"type\":\"ConnectorPlacement.EquallySpacedRectSide\",\"uuid\":\"6b3cab93-b4c4-4362-9fab-fb0578b34e5e\"},{\"content\":{\"side\":\"BOTTOM\"},\"type\":\"ConnectorPlacement.EquallySpacedRectSide\",\"uuid\":\"096b815e-5cad-442a-9b00-3e24e5e9ca79\"}]},\"type\":\"ConnectorPlacement.EquallySpacedConnector\",\"uuid\":\"7d9f7809-5a51-462b-83e3-36dfed501a9a\"}],\"packageUris\":[\"http://schema.mathworks.com/mf0/Connector/R2020b\"],\"version\":\"1.0\"}"
      mask Display: image('$imagefile'); % Use "Edit Image" on toolstrip to change.
  Motor 3 : Subsystem
      settings: PortSchema="{\"entries\":[{\"content\":{\"sides\":[{\"content\":{},\"type\":\"ConnectorPlacement.EquallySpacedRectSide\",\"uuid\":\"be0e671a-e613-444c-b8e2-6f7a2adfd701\"},{\"content\":{\"side\":\"RIGHT\"},\"type\":\"ConnectorPlacement.EquallySpacedRectSide\",\"uuid\":\"98a92d25-e065-434b-83fd-1db07c9786c9\"},{\"content\":{\"connectorIds\":[\"LConn1\"],\"side\":\"TOP\"},\"type\":\"ConnectorPlacement.EquallySpacedRectSide\",\"uuid\":\"6b3cab93-b4c4-4362-9fab-fb0578b34e5e\"},{\"content\":{\"connectorIds\":[\"RConn1\"],\"side\":\"BOTTOM\"},\"type\":\"ConnectorPlacement.EquallySpacedRectSide\",\"uuid\":\"096b815e-5cad-442a-9b00-3e24e5e9ca79\"}]},\"type\":\"ConnectorPlacement.EquallySpacedConnector\",\"uuid\":\"7d9f7809-5a51-462b-83e3-36dfed501a9a\"}],\"packageUris\":[\"http://schema.mathworks.com/mf0/Connector/R2020b\"],\"version\":\"1.0\"}"
      mask Display: image('$imagefile'); % Use "Edit Image" on toolstrip to change.
  Motor 4 : Subsystem
      settings: PortSchema="{\"entries\":[{\"content\":{\"sides\":[{\"content\":{},\"type\":\"ConnectorPlacement.EquallySpacedRectSide\",\"uuid\":\"be0e671a-e613-444c-b8e2-6f7a2adfd701\"},{\"content\":{\"side\":\"RIGHT\"},\"type\":\"ConnectorPlacement.EquallySpacedRectSide\",\"uuid\":\"98a92d25-e065-434b-83fd-1db07c9786c9\"},{\"content\":{\"connectorIds\":[\"LConn1\"],\"side\":\"TOP\"},\"type\":\"ConnectorPlacement.EquallySpacedRectSide\",\"uuid\":\"6b3cab93-b4c4-4362-9fab-fb0578b34e5e\"},{\"content\":{\"connectorIds\":[\"RConn1\"],\"side\":\"BOTTOM\"},\"type\":\"ConnectorPlacement.EquallySpacedRectSide\",\"uuid\":\"096b815e-5cad-442a-9b00-3e24e5e9ca79\"}]},\"type\":\"ConnectorPlacement.EquallySpacedConnector\",\"uuid\":\"7d9f7809-5a51-462b-83e3-36dfed501a9a\"}],\"packageUris\":[\"http://schema.mathworks.com/mf0/Connector/R2020b\"],\"version\":\"1.0\"}"
      mask Display: image('$imagefile'); % Use "Edit Image" on toolstrip to change.
  Motor 5 : Subsystem
      settings: PortSchema="{\"entries\":[{\"content\":{\"sides\":[{\"content\":{},\"type\":\"ConnectorPlacement.EquallySpacedRectSide\",\"uuid\":\"be0e671a-e613-444c-b8e2-6f7a2adfd701\"},{\"content\":{\"side\":\"RIGHT\"},\"type\":\"ConnectorPlacement.EquallySpacedRectSide\",\"uuid\":\"98a92d25-e065-434b-83fd-1db07c9786c9\"},{\"content\":{\"connectorIds\":[\"LConn1\"],\"side\":\"TOP\"},\"type\":\"ConnectorPlacement.EquallySpacedRectSide\",\"uuid\":\"6b3cab93-b4c4-4362-9fab-fb0578b34e5e\"},{\"content\":{\"connectorIds\":[\"RConn1\"],\"side\":\"BOTTOM\"},\"type\":\"ConnectorPlacement.EquallySpacedRectSide\",\"uuid\":\"096b815e-5cad-442a-9b00-3e24e5e9ca79\"}]},\"type\":\"ConnectorPlacement.EquallySpacedConnector\",\"uuid\":\"7d9f7809-5a51-462b-83e3-36dfed501a9a\"}],\"packageUris\":[\"http://schema.mathworks.com/mf0/Connector/R2020b\"],\"version\":\"1.0\"}"
      mask Display: image('$imagefile'); % Use "Edit Image" on toolstrip to change.
  Motor 6 : Subsystem
      settings: PortSchema="{\"entries\":[{\"content\":{\"sides\":[{\"content\":{},\"type\":\"ConnectorPlacement.EquallySpacedRectSide\",\"uuid\":\"be0e671a-e613-444c-b8e2-6f7a2adfd701\"},{\"content\":{\"side\":\"RIGHT\"},\"type\":\"ConnectorPlacement.EquallySpacedRectSide\",\"uuid\":\"98a92d25-e065-434b-83fd-1db07c9786c9\"},{\"content\":{\"connectorIds\":[\"LConn1\"],\"side\":\"TOP\"},\"type\":\"ConnectorPlacement.EquallySpacedRectSide\",\"uuid\":\"6b3cab93-b4c4-4362-9fab-fb0578b34e5e\"},{\"content\":{\"connectorIds\":[\"RConn1\"],\"side\":\"BOTTOM\"},\"type\":\"ConnectorPlacement.EquallySpacedRectSide\",\"uuid\":\"096b815e-5cad-442a-9b00-3e24e5e9ca79\"}]},\"type\":\"ConnectorPlacement.EquallySpacedConnector\",\"uuid\":\"7d9f7809-5a51-462b-83e3-36dfed501a9a\"}],\"packageUris\":[\"http://schema.mathworks.com/mf0/Connector/R2020b\"],\"version\":\"1.0\"}"
      mask Display: image('$imagefile'); % Use "Edit Image" on toolstrip to change.
  PS-Simulink Converter{,1..3} (4 alike) : nesl_utility/PS-Simulink Converter  PhysicalDomain=network_engine_domain  SubClassName=ps_output  LeftPortType=input  RightPortType=output  PseudoPeriodic=off  Frequencies=[]  Unit=inherit  AffineConversion=off
  Scope : Scope  NumInputPorts=2
  Scope1 : Scope  NumInputPorts=2
  Solver Configuration1 : nesl_utility/Solver Configuration  PhysicalDomain=network_engine_domain  SubClassName=solver  LeftPortType=input  RightPortType=generic  Tones=[]  Harmonics=[]  SimulateNoise=off  Profile=off  UseLocalSampling=off  EnableSwitchedLinearOptims=on  FrequencyDomain=off  UseCCode=off  RelTol=0.001  AbsTol=0.001  MinStep=1e-09  ToWorkspace=off  RevertToSquareIcSolve=off  NumHomotopyIterations=100  PhasorMode=off  PhasorModeNumHarmonics=1  DoDC=off  ResidualTolerance=1e-09  UseLocalSolver=off  LocalSolverChoice=NE_BACKWARD_EULER_ADVANCER  LocalSolverSampleTime=0.001  DoFixedCost=off  MaxNonlinIter=3  MaxModeIter=2  LinearAlgebra=auto  EquationFormulation=NE_TIME_EF  DelaysMemoryBudget=1024  AutomaticFiltering=on  FilteringTimeConstant=0.001  PartitionStorageMethod=AS_NEEDED  PartitionMemoryBudget=1024  PartitionMethod=ROBUST
  Subsystem : Subsystem
  Subsystem1 : Subsystem
  Transfer Fcn{1..4} (4 alike) : TransferFcn  Numerator=[1*2*pi]  Denominator=[1 1*2*pi]
  Voltage Sensor : fl_lib/Electrical/Electrical Sensors/Voltage Sensor
  Voltage Sensor1 : fl_lib/Electrical/Electrical Sensors/Voltage Sensor
  tag scope: BatteryVoltage1=global, BatteryVoltage2=global, I_ESC_IN_1=global, I_ESC_IN_2=global
  wires:
  PS-Simulink Converter/1 -> Transfer Fcn2/1
  PS-Simulink Converter1/1 -> Transfer Fcn1/1
  PS-Simulink Converter3/1 -> Transfer Fcn3/1
  PS-Simulink Converter2/1 -> Transfer Fcn4/1
  Transfer Fcn2/1 -> Scope/1, [I_ESC_IN_1], Subsystem/1(In1)  "1"
  Transfer Fcn1/1 -> Scope/2, Subsystem1/1(In1), [I_ESC_IN_2]  "2"
  Transfer Fcn3/1 -> Scope1/2, [BatteryVoltage2]
  Transfer Fcn4/1 -> Scope1/1, Display/1, [BatteryVoltage1]
  connections:
  Motor 4/LConn1 -- Motor 2/LConn2 -- Current Sensor 2/RConn2 -- Motor 6/LConn1
  Motor 5/RConn1 -- Motor 3/LConn1 -- Solver Configuration1/RConn1 -- Voltage Sensor1/RConn2 -- Battery 2 (Model based)/RConn2 -- Motor 6/RConn1 -- Motor 2/LConn1 -- Motor 4/RConn1 -- Ground/LConn1 -- Battery 1 (Model based)/RConn2 -- Voltage Sensor/RConn2 -- Motor 1/LConn1
  PS-Simulink Converter/LConn1 -- Current Sensor 1/RConn1
  Motor 1/RConn1 -- Motor 3/RConn1 -- Current Sensor 1/RConn2
  PS-Simulink Converter1/LConn1 -- Current Sensor 2/RConn1
  Current Sensor 1/LConn1 -- Voltage Sensor/LConn1 -- Battery 1 (Model based)/LConn1 -- Motor 5/LConn1
  Voltage Sensor1/LConn1 -- Current Sensor 2/LConn1 -- Battery 2 (Model based)/LConn1
  PS-Simulink Converter2/LConn1 -- Voltage Sensor/RConn1
  PS-Simulink Converter3/LConn1 -- Voltage Sensor1/RConn1
  Battery 2 (Model based)/RConn1 -- Subsystem1/RConn1
  Battery 1 (Model based)/RConn1 -- Subsystem/RConn1

== system Drone_Simulation/PLANT MODEL/ENVIRONMENT ==
  Ground : Subsystem  mask{rhoE=1000000, rgbE=[0 0.7 0.1], opE=1}
      mask prompts: rhoE "Density of Ground (kg/m^3)"; rgbE "Color of Ground [R G B]"; opE "Opacity of Ground (0-1)"
      mask Display: image('$imagefile'); % Use "Edit Image" on toolstrip to change.
  Sky : Subsystem  mask{rhoS=0.000001, rgbS=[0.529 0.808 0.922], opS=0.5}
      mask prompts: rhoS "Density of Sky (kg/m^3)"; rgbS "Color of Sky [R G B]"; opS "Opacity of Sky (0-1)"
      mask Display: image('$imagefile'); % Use "Edit Image" on toolstrip to change.
  World Frame : sm_lib/Frames and Transforms/World Frame
  GC : PMIOPort  Side=Left
  World Frame1 : PMIOPort  Port=2  Side=Right
  connections:
  World Frame/RConn1 -- Sky/RConn1 -- Ground/RConn1 -- World Frame1/RConn1
  Ground/LConn1 -- GC/RConn1

== system Drone_Simulation/PLANT MODEL/PROPELLER AND ARMS ==
  Arms : Subsystem  mask{rho1=1518, rgb1=[0.753 0.753 0.753], op1=1, rhoM=14013}
      mask prompts: rho1 "Density of Arm (kg/m^3)"; rgb1 "Color of Arm [R G B]"; op1 "Opacity of Arm (0-1)"; rhoM "Density of Motors"
      mask Display: image('Arm.jpg'); % Use "Edit Image" on toolstrip to change.
  Propellers Thurst and Torque : Subsystem  mask{rhoP=2649, rgbP=[1 0.549 0.2], opP=1}
      mask prompts: rhoP "Density of Propeller (kg/m^3)"; rgbP "Color of Propeller [R G B]"; opP "Opacity of Propeller (0-1)"
      mask Display: image('$imagefile'); % Use "Edit Image" on toolstrip to change.
  Fuselage : PMIOPort  Side=Right
  Left Contact Force : PMIOPort  Port=2  Side=Right
  Right Contact Force : PMIOPort  Port=3  Side=Right
  connections:
  Arms/LConn4 -- Propellers Thurst and Torque/RConn4
  Arms/LConn7 -- Fuselage/RConn1
  Arms/RConn1 -- Left Contact Force/RConn1
  Arms/RConn2 -- Right Contact Force/RConn1
  Arms/LConn5 -- Propellers Thurst and Torque/RConn5
  Arms/LConn6 -- Propellers Thurst and Torque/RConn6
  Arms/LConn3 -- Propellers Thurst and Torque/RConn3
  Arms/LConn2 -- Propellers Thurst and Torque/RConn2
  Arms/LConn1 -- Propellers Thurst and Torque/RConn1

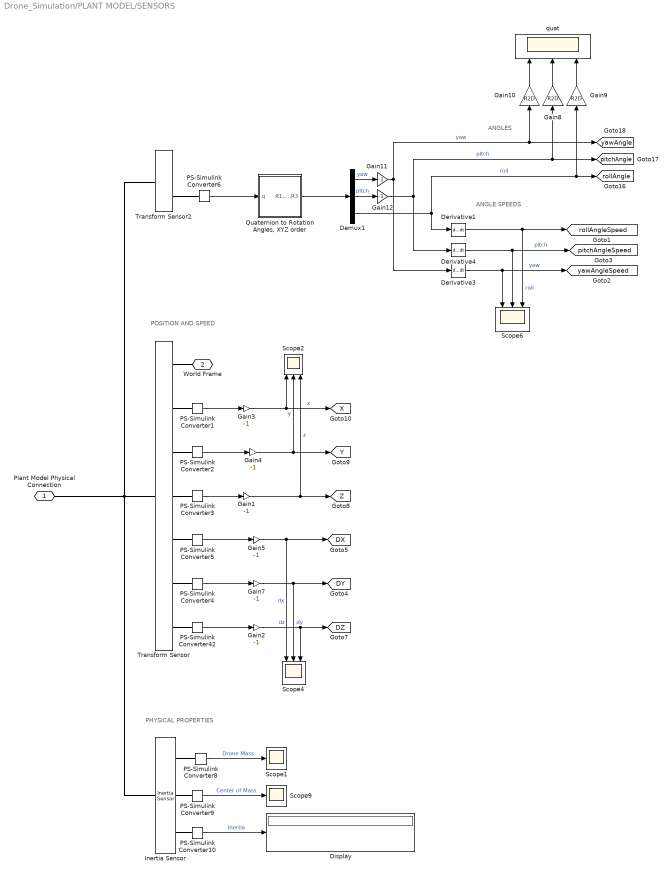
== system Drone_Simulation/PLANT MODEL/SENSORS ==
  note: POSITION AND SPEED
  note: PHYSICAL PROPERTIES
  note: ANGLE SPEEDS
  note: ANGLES
  Demux1 : Demux  Outputs=3
  Derivative1 : Derivative  CoefficientInTFapproximation=1e-9
  Derivative3 : Derivative  CoefficientInTFapproximation=1e-9
  Derivative4 : Derivative  CoefficientInTFapproximation=1e-9
  Display : Display
  Gain{1..5,7,11..12} (8 alike) : Gain  Gain=-1
  Gain10 : Gain  Gain=R2D
  Gain8 : Gain  Gain=R2D
  Gain9 : Gain  Gain=R2D
  Inertia Sensor : sm_lib/Body Elements/Inertia Sensor  SensorExtent=BodyGroup  SpanWeldJoints=off  ExcludeGroundedBodies=off  MeasurementFrame=Attached  SenseMass=on  SenseCenterOfMass=on  SenseInertiaMatrix=on  SenseCenteredInertiaMatrix=off  SensePrincipalInertiaMatrix=off  SenseRotationMatrix=off  GraphicType=None  PrincipalInertiaFrameSize=20  GraphicVisPropType=SimpleVisualProperties  GraphicDiffuseColor=[0.5 0.5 0.5]  GraphicSpecularColor=[0.5 0.5 0.5 1.0]  GraphicAmbientColor=[0.15 0.15 0.15 1.0]  GraphicEmissiveColor=[0.0 0.0 0.0 1.0]  GraphicShininess=75  GraphicOpacity=1.0
      settings: SourceProductBaseCode=MS
  PS-Simulink Converter{1..6,8..9,42} (9 alike) : nesl_utility/PS-Simulink Converter  PhysicalDomain=network_engine_domain  SubClassName=ps_output  LeftPortType=input  RightPortType=output  PseudoPeriodic=off  Frequencies=[]  Unit=inherit  AffineConversion=off
  PS-Simulink Converter10 : nesl_utility/PS-Simulink Converter  PhysicalDomain=network_engine_domain  SubClassName=ps_output  LeftPortType=input  RightPortType=output  PseudoPeriodic=off  Frequencies=[]  Unit=inherit  AffineConversion=on
  "Quaternion to Rotation Angles, XYZ order" : Subsystem
  Scope1 : Scope
  Scope2 : Scope  NumInputPorts=3
  Scope4 : Scope  NumInputPorts=3
  Scope6 : Scope  NumInputPorts=3
  Scope9 : Scope
  Transform Sensor : sm_lib/Frames and Transforms/Transform Sensor  MeasurementFrame=World  SenseAngle=off  SenseAxis=off  SenseAngle1=off  SenseAngle2=off  SenseAngle3=off  SenseQ=off  SenseR=off  SenseOmegaX=off  SenseOmegaY=off  SenseOmegaZ=off  SenseOmega1=off  SenseOmega2=off  SenseOmega3=off  SenseQDot=off  SenseRDot=off  SenseAlphaX=off  SenseAlphaY=off  SenseAlphaZ=off  SenseAlpha1=off  SenseAlpha2=off  SenseAlpha3=off  SenseQDDot=off  SenseRDDot=off  SenseX=on  SenseY=on  SenseZ=on  SenseRad=off  SenseAzim=off  SenseDist=off  SenseInc=off  SenseXDot=on  SenseYDot=on  SenseZDot=on  SenseRadDot=off  SenseAzimDot=off  SenseDistDot=off  SenseIncDot=off  SenseXDDot=off  SenseYDDot=off  SenseZDDot=off  SenseRadDDot=off  SenseAzimDDot=off  SenseDistDDot=off  SenseIncDDot=off
  Transform Sensor2 : sm_lib/Frames and Transforms/Transform Sensor  MeasurementFrame=World  SenseAngle=off  SenseAxis=off  SenseAngle1=off  SenseAngle2=off  SenseAngle3=off  SenseQ=on  SenseR=off  SenseOmegaX=off  SenseOmegaY=off  SenseOmegaZ=off  SenseOmega1=off  SenseOmega2=off  SenseOmega3=off  SenseQDot=off  SenseRDot=off  SenseAlphaX=off  SenseAlphaY=off  SenseAlphaZ=off  SenseAlpha1=off  SenseAlpha2=off  SenseAlpha3=off  SenseQDDot=off  SenseRDDot=off  SenseX=off  SenseY=off  SenseZ=off  SenseRad=off  SenseAzim=off  SenseDist=off  SenseInc=off  SenseXDot=off  SenseYDot=off  SenseZDot=off  SenseRadDot=off  SenseAzimDot=off  SenseDistDot=off  SenseIncDot=off  SenseXDDot=off  SenseYDDot=off  SenseZDDot=off  SenseRadDDot=off  SenseAzimDDot=off  SenseDistDDot=off  SenseIncDDot=off
  quat : Scope  NumInputPorts=3
  Plant Model Physical Connection : PMIOPort  Side=Right
  World Frame : PMIOPort  Port=2  Side=Right
  tag scope: DX=global, DY=global, DZ=global, X=global, Y=global, Z=global, pitchAngle=global, pitchAngleSpeed=global, rollAngle=global, rollAngleSpeed=global, yawAngle=global, yawAngleSpeed=global
  wires:
  PS-Simulink Converter9/1 -> Scope9/1  "Center of Mass"
  PS-Simulink Converter8/1 -> Scope1/1  "Drone Mass"
  PS-Simulink Converter42/1 -> Gain2/1
  PS-Simulink Converter1/1 -> Gain3/1
  PS-Simulink Converter3/1 -> Gain1/1
  PS-Simulink Converter2/1 -> Gain4/1
  Gain2/1 -> Scope4/3, [DZ]  "dz"
  Gain1/1 -> [Z], Scope2/3  "z"
  PS-Simulink Converter4/1 -> Gain7/1
  PS-Simulink Converter5/1 -> Gain5/1
  Gain3/1 -> Scope2/1, [X]  "x"
  Gain4/1 -> [Y], Scope2/2  "y"
  Gain5/1 -> [DX], Scope4/1  "dx"
  Gain7/1 -> [DY], Scope4/2  "dy"
  Gain12/1 -> [pitchAngle], Gain8/1, Derivative4/1  "pitch"
  Demux1/3 -> [rollAngle], Gain9/1, Derivative1/1  "roll"
  Demux1/2 -> Gain12/1  "pitch"
  Demux1/1 -> Gain11/1  "yaw"
  "Quaternion to Rotation Angles, XYZ order"/1(R1,R2,R3) -> Demux1/1
  PS-Simulink Converter6/1 -> "Quaternion to Rotation Angles, XYZ order"/1(q)
  Gain10/1 -> quat/1
  Gain8/1 -> quat/2
  Gain9/1 -> quat/3
  Derivative3/1 -> [yawAngleSpeed], Scope6/1  "yaw"
  Derivative4/1 -> [pitchAngleSpeed], Scope6/2  "pitch"
  Derivative1/1 -> [rollAngleSpeed], Scope6/3  "roll"
  Gain11/1 -> [yawAngle], Gain10/1, Derivative3/1  "yaw"
  PS-Simulink Converter10/1 -> Display/1  "Inertia"
  connections:
  PS-Simulink Converter8/LConn1 -- Inertia Sensor/RConn1
  PS-Simulink Converter9/LConn1 -- Inertia Sensor/RConn2
  PS-Simulink Converter10/LConn1 -- Inertia Sensor/RConn3
  Plant Model Physical Connection/RConn1 -- Transform Sensor2/LConn1 -- Transform Sensor/LConn1 -- Inertia Sensor/LConn1
  World Frame/RConn1 -- Transform Sensor/RConn1
  PS-Simulink Converter6/LConn1 -- Transform Sensor2/RConn2
  PS-Simulink Converter1/LConn1 -- Transform Sensor/RConn2
  PS-Simulink Converter3/LConn1 -- Transform Sensor/RConn4
  PS-Simulink Converter2/LConn1 -- Transform Sensor/RConn3
  PS-Simulink Converter5/LConn1 -- Transform Sensor/RConn5
  PS-Simulink Converter4/LConn1 -- Transform Sensor/RConn6
  PS-Simulink Converter42/LConn1 -- Transform Sensor/RConn7

== system Drone_Simulation/CONTROL ALLOCATION/Inputs Needed For Reliability Model/Subsystem ==
  In1 : Inport
  In2 : Inport  Port=2
  Gain5 : Gain  Gain=Re
  Gain6 : Gain  Gain=1/Ub
  Sum5 : Sum
  Out1 : Outport
  wires:
  Sum5/1 -> Gain6/1  "Ueo"
  Gain5/1 -> Sum5/2
  In1/1 -> Sum5/1
  Gain6/1 -> Out1/1
  In2/1 -> Gain5/1

== system Drone_Simulation/CONTROL ALLOCATION/Inputs Needed For Reliability Model/Subsystem1 ==
  In1 : Inport
  In2 : Inport  Port=2
  ESC Output Voltage : Constant  Value=5
  Product : Product  Inputs=3
  Out1 : Outport
  wires:
  ESC Output Voltage/1 -> Product/3
  In2/1 -> Product/2
  Product/1 -> Out1/1
  In1/1 -> Product/1

== system Drone_Simulation/CONTROL ALLOCATION/Reliability Observer (BNG)1/Failure Prediction Model ==
  N (RPM) : Inport
  M (Nm) : Inport  Port=2
  Constant2 : Constant  Value=pconst
  Gain : Gain  Gain=pi/180
  Power : Math  Operator=pow  SaturateOnIntegerOverflow=on
  Product10 : Product
  q (N^3.m^3/s) : Outport
  wires:
  Gain/1 -> Product10/1
  N (RPM)/1 -> Gain/1
  Product10/1 -> q (N^3.m^3/s)/1  "q (N^3.m^3/s)"
  M (Nm)/1 -> Power/1
  Power/1 -> Product10/2
  Constant2/1 -> Power/2

== system Drone_Simulation/CONTROL ALLOCATION/Reliability Observer (BNG)1/Realtime Reliability Observer (BNG) ==
  q (N^3.m^3/s) : Inport
  Constant10 : Constant  Value=bBNG-1
  Constant11 : Constant  Value=bBNG
  Constant4 : Constant  Value=0.2426
  Constant5 : Constant  Value=1.243
  Constant6 : Constant  Value=RrefBNG
  Constant7 : Constant  Value=bBNG
  Constant8 : Constant  Value=bBNG
  Constant9 : Constant  Value=pconst
  Divide : Product  Inputs=*/
  Exp : Math  SaturateOnIntegerOverflow=on
  Gain : Gain  Gain=-1
  Gain1 : Gain  Gain=-1
  Integrator : Integrator  InitialConditionSource=external  InitialCondition=[0;0;0;0;0;0]
  Motors Reliability Initial Condition : Constant  Value=[BNG_Motor1,BNG_Motor2,BNG_Motor3,BNG_Motor4,BNG_Motor5,BNG_Motor6]
  Power{1..4} (4 alike) : Math  Operator=pow  SaturateOnIntegerOverflow=on
  Product1 : Product
  Product2 : Product  Inputs=/*
  Product3 : Product  Inputs=/*
  Product4 : Product  Inputs=*/
  Product5 : Product
  Reciprocal : Product  Inputs=/
  Terminator : Terminator
  ln : Math  Operator=log  SaturateOnIntegerOverflow=on
  theta_Q : Constant  Value=25
  Lambda : Outport
  R : Outport  Port=2
  wires:
  Divide/1 -> Integrator/2
  Motors Reliability Initial Condition/1 -> Divide/1
  Reciprocal/1 -> Power1/2
  Constant7/1 -> Reciprocal/1
  Exp/1 -> R/1  "R"
  Product2/1 -> Terminator/1  "theta_Q"
  Gain1/1 -> Power1/1
  q (N^3.m^3/s)/1 -> Integrator/1
  Constant6/1 -> ln/1
  Constant11/1 -> Power4/2
  Product5/1 -> Lambda/1  "Lambda"
  Gain/1 -> Exp/1
  Constant8/1 -> Product3/2
  Product3/1 -> Product5/2
  Product1/1 -> Product2/2, Divide/2  "Q_10 (N^3.m^3/s)"
  Power4/1 -> Gain/1
  Constant10/1 -> Power3/2
  theta_Q/1 -> Product3/1, Product4/2
  Constant9/1 -> Power2/2
  Product4/1 -> Power3/1, Power4/1
  Power2/1 -> Product1/2
  Constant5/1 -> Power2/1
  Power1/1 -> Product2/1
  Constant4/1 -> Product1/1
  ln/1 -> Gain1/1
  Integrator/1 -> Product4/1  "Q (N^3.m^3)"
  Power3/1 -> Product5/1

== system Drone_Simulation/CONTROL ALLOCATION/Reliability Observer (CAPEV)1/Cumulative Aging EVCAP ==
  In1 : Inport
  In3 : Inport  Port=2
  Aging Velocity : Product
  Cumulative Aging : Integrator  InitialConditionSource=external
  Display{,1..8} (9 alike) : Display
  Divide : Product  Inputs=**
  Divide2 : Product  Inputs=/*/
  Divide4 : Product  Inputs=*/
  EaEVCAP1 : Constant  Value=EaEVCAP
  K1 : Constant  Value=k_b
  Math Function1 : Math  SaturateOnIntegerOverflow=on
  Math Function8 : Math  Operator=pow  SaturateOnIntegerOverflow=on
  Motors Reliability Initial Condition : Constant  Value=[CAPEV_Motor1,CAPEV_Motor2,CAPEV_Motor3,CAPEV_Motor4,CAPEV_Motor5,CAPEV_Motor6]
  Unary Minus : UnaryMinus
  VmaxEVCAP : Constant  Value=VmaxEVCAP
  nEVCAP : Constant  Value=nEVCAP
  Out1 : Outport
  wires:
  [VrefEVCAP] -> Display8/1, Divide/2
  Divide/1 -> Display/1, Cumulative Aging/2
  Motors Reliability Initial Condition/1 -> Divide/1
  In3/1 -> Divide2/1, Display7/1
  Cumulative Aging/1 -> Out1/1
  Divide2/1 -> Math Function1/1
  EaEVCAP1/1 -> Unary Minus/1, Display6/1
  Math Function8/1 -> Aging Velocity/1, Display2/1
  Aging Velocity/1 -> Cumulative Aging/1, Display3/1
  VmaxEVCAP/1 -> Divide4/2
  Unary Minus/1 -> Divide2/2
  nEVCAP/1 -> Math Function8/2
  Divide4/1 -> Math Function8/1, Display1/1
  In1/1 -> Divide4/1
  Math Function1/1 -> Aging Velocity/2, Display4/1
  K1/1 -> Divide2/3, Display5/1

== system Drone_Simulation/CONTROL ALLOCATION/Reliability Observer (CAPEV)1/LambdaEV ==
  In1 : Inport
  In2 : Inport  Port=2
  In3 : Inport  Port=3
  Bias : Bias  Bias=-1
  Divide : Product  Inputs=*/
  Divide1 : Product  Inputs=**/
  Math Function : Math  Operator=pow  SaturateOnIntegerOverflow=on
  bEVCAP : Constant  Value=bEVCAP
  Out1 : Outport
  wires:
  Bias/1 -> Math Function/2
  Math Function/1 -> Divide1/1
  bEVCAP/1 -> Bias/1, Divide1/2
  Divide1/1 -> Out1/1
  In2/1 -> Divide/2
  In1/1 -> Divide/1
  In3/1 -> Divide1/3
  Divide/1 -> Math Function/1

== system Drone_Simulation/CONTROL ALLOCATION/Reliability Observer (CAPEV)1/ReliabilityEVCAP ==
  In1 : Inport
  In2 : Inport  Port=2
  Abs : Abs
  Divide6 : Product  Inputs=*//
  Math Function4 : Math  Operator=log  SaturateOnIntegerOverflow=on
  Math Function5 : Math  Operator=reciprocal  SaturateOnIntegerOverflow=on
  Math Function6 : Math  Operator=pow  SaturateOnIntegerOverflow=on
  Math Function7 : Math  Operator=pow  SaturateOnIntegerOverflow=on
  R(V) : Math  SaturateOnIntegerOverflow=on
  RrefEVCAP : Constant  Value=RrefEVCAP
  Unary Minus2 : UnaryMinus
  Unary Minus3 : UnaryMinus
  bEVCAP1 : Constant  Value=bEVCAP
  bEVCAP2 : Constant  Value=bEVCAP
  Out1 : Outport
  wires:
  bEVCAP1/1 -> Unary Minus2/1
  Math Function5/1 -> Math Function6/2
  In1/1 -> Divide6/1
  Math Function6/1 -> Divide6/3
  Divide6/1 -> Math Function7/1
  Unary Minus3/1 -> R(V)/1
  Math Function4/1 -> Abs/1
  Unary Minus2/1 -> Math Function5/1
  RrefEVCAP/1 -> Math Function4/1
  R(V)/1 -> Out1/1
  Math Function7/1 -> Unary Minus3/1
  Abs/1 -> Math Function6/1
  bEVCAP2/1 -> Math Function7/2
  In2/1 -> Divide6/2

== system Drone_Simulation/CONTROL ALLOCATION/Reliability Observer (CAPEV)1/VrefEVCAP ==
  Divide3 : Product  Inputs=*/
  Divide5 : Product  Inputs=*//
  EaEVCAP : Constant  Value=EaEVCAP
  K : Constant  Value=k_b
  LnomEVCAP : Constant  Value=LnomEVCAP
  Math Function2 : Math  Operator=pow  SaturateOnIntegerOverflow=on
  Math Function3 : Math  SaturateOnIntegerOverflow=on
  TrefEVCAP : Constant  Value=TrefEVCAP
  Unary Minus1 : UnaryMinus
  VmaxEVCAP1 : Constant  Value=VmaxEVCAP
  VnomEVCAP : Constant  Value=VnomEVCAP
  Vref : Product  Inputs=3
  nEVCAP1 : Constant  Value=nEVCAP
  Out1 : Outport
  tag scope: VrefEVCAP=global
  wires:
  nEVCAP1/1 -> Math Function2/2
  VnomEVCAP/1 -> Divide3/1
  Divide3/1 -> Math Function2/1
  Vref/1 -> Out1/1, [VrefEVCAP]
  TrefEVCAP/1 -> Divide5/3
  Divide5/1 -> Math Function3/1
  Unary Minus1/1 -> Divide5/1
  VmaxEVCAP1/1 -> Divide3/2
  Math Function3/1 -> Vref/3
  K/1 -> Divide5/2
  EaEVCAP/1 -> Unary Minus1/1
  LnomEVCAP/1 -> Vref/1
  Math Function2/1 -> Vref/2
